simulink model "gm_PF"  (R2015a)
settings: Solver=FixedStepDiscrete  SolverMode=SingleTasking  StartTime=0.0  StopTime=2  RelTol=1e-3
libraries: dspsrcs4 x3, dspsnks4 x1
settings Model: Creator=aluno  LastModifiedBy=aluno
settings DataIOCC: SaveOutput=off  SaveTime=off
settings OptimizationCC: BlockReduction=off  ConditionallyExecuteInputs=off  InlineParams=on
settings DebuggingCC: AlgebraicLoopMsg=error  InheritedTsInSrcMsg=none  SingleTaskRateTransMsg=error  StrictBusMsg=ErrorOnBusTreatedAsVector
settings HardwareCC: ProdHWDeviceType=ASIC/FPGA->ASIC/FPGA  ProdEqTarget=off

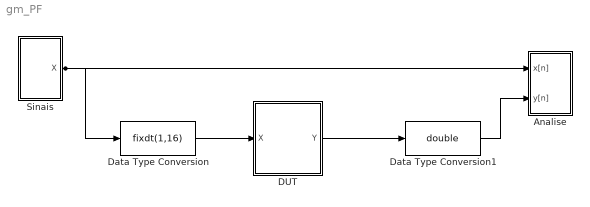
== system gm_PF ==
  Analise : Subsystem
  DUT : Subsystem
  Data Type Conversion : DataTypeConversion  OutMin=-1  OutMax=0.99  OutDataTypeStr=fixdt(1,16)
  Data Type Conversion1 : DataTypeConversion  OutDataTypeStr=double
  Sinais : Subsystem  mask{fa=8000, spf=1, fonte=2, v1=0.5, f1=1000, tchirp=2}
      mask prompts: fa "Freq. amostragem (Hz)"; spf "Amostras por frame"; fonte "Fonte (switch)"; v1 "Amplitude da senoide"; f1 "Freq. da senoide"; tchirp "Tempo Chirp"
      mask TypeOptions fonte: 1 | 2 | 3 | 4 | 5
  wires:
  Data Type Conversion1/1 -> Analise/2(y[n])
  Data Type Conversion/1 -> DUT/1(X)
  DUT/1(Y) -> Data Type Conversion1/1
  Sinais/1(X) -> Data Type Conversion/1, Analise/1(x[n])

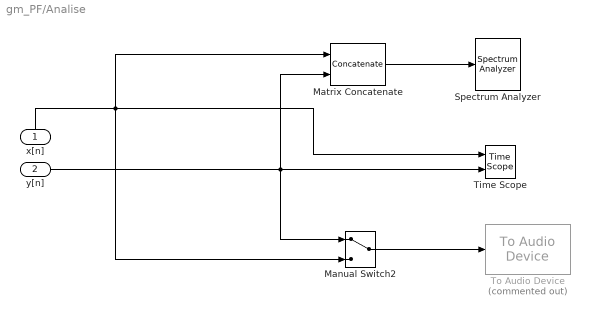
== system gm_PF/Analise ==
  x[n] : Inport
  y[n] : Inport  Port=2
  Manual Switch2 : ManualSwitch
  Matrix Concatenate : Concatenate  Mode=Multidimensional array  ConcatenateDimension=2
  Spectrum Analyzer : SpectrumAnalyzer
  Time Scope : TimeScope  DefaultConfigurationName=spbscopes.TimeScopeBlockCfg  NumInputPorts=2
  To Audio Device : dspsnks4/To Audio Device  Commented=on  deviceName=Default  inheritSampleRate=on  sampleRate=44100  deviceDatatype=Determine from input data type  autoBufferSize=on  bufferSize=4096  queueDuration=1.0  defaultOutputChannelMapping=on  outputChannelMapping=1:2  outputNumUnderrunSamples=off
  wires:
  Manual Switch2/1 -> To Audio Device/1
  y[n]/1 -> Time Scope/2, Matrix Concatenate/2, Manual Switch2/1
  x[n]/1 -> Matrix Concatenate/1, Time Scope/1, Manual Switch2/2
  Matrix Concatenate/1 -> Spectrum Analyzer/1

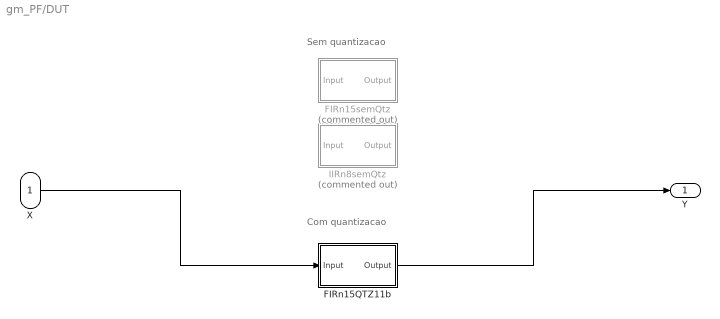
== system gm_PF/DUT ==
  note: Sem quantizacao
  note: Com quantizacao
  X : Inport
  FIRn15QTZ11b : Subsystem  Tag=FilterWizardSubSystem
      settings: ErrorFcn=dspFilterRealizedInBasicElemsAlgLoopErrFcnCallback
  FIRn15semQtz : Subsystem  Tag=FilterWizardSubSystem  Commented=on
      settings: ErrorFcn=dspFilterRealizedInBasicElemsAlgLoopErrFcnCallback
  IIRn8semQtz : Subsystem  Tag=FilterWizardSubSystem  Commented=on
      settings: ErrorFcn=dspFilterRealizedInBasicElemsAlgLoopErrFcnCallback
  Y : Outport
  wires:
  FIRn15QTZ11b/1(Output) -> Y/1
  X/1 -> FIRn15QTZ11b/1(Input)

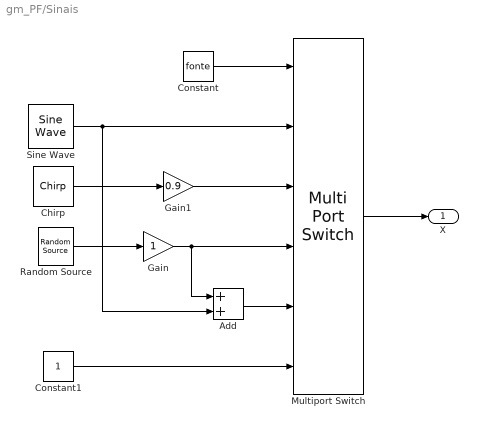
== system gm_PF/Sinais ==
  Add : Sum
  Chirp : dspsrcs4/Chirp  sweep=Linear  mode=Unidirectional  f0=1  f1=fa/2  t1=tchirp  Tsweep=tchirp  phase=0  Ts=1/fa  spf=spf  datatype=Double
  Constant : Constant  Value=fonte
  Constant1 : Constant
  Gain : Gain
  Gain1 : Gain  Gain=0.9
  Multiport Switch : MultiPortSwitch  Inputs=5
  Random Source : dspsrcs4/Random Source  SrcType=Uniform  NormMethod=Ziggurat  CltLength=12  MinVal=-1  MaxVal=1  MeanVal=0  VarVal=1  RepMode=Not repeatable  rawSeed=1  IsInherit=off  SampMode=Discrete  SampTime=1/fa  SampFrame=spf  DataType=Double  OutComplex=Real
  Sine Wave : dspsrcs4/Sine Wave  Amplitude=v1  Frequency=f1  Phase=0  SampleMode=Discrete  OutComplex=Real  CompMethod=Trigonometric fcn  TableSize=Speed  SampleTime=1/fa  SamplesPerFrame=spf  ResetState=Restart at time zero  dataType=double  wordLen=16  udDataType=sfix(16)  fracBitsMode=Best precision  numFracBits=15  OutDataTypeStr=double  LastOutDataTypeStr=double
  X : Outport
  wires:
  Gain1/1 -> Multiport Switch/3
  Random Source/1 -> Gain/1
  Constant1/1 -> Multiport Switch/6
  Add/1 -> Multiport Switch/5
  Constant/1 -> Multiport Switch/1
  Multiport Switch/1 -> X/1
  Sine Wave/1 -> Multiport Switch/2, Add/2
  Chirp/1 -> Gain1/1
  Gain/1 -> Multiport Switch/4, Add/1

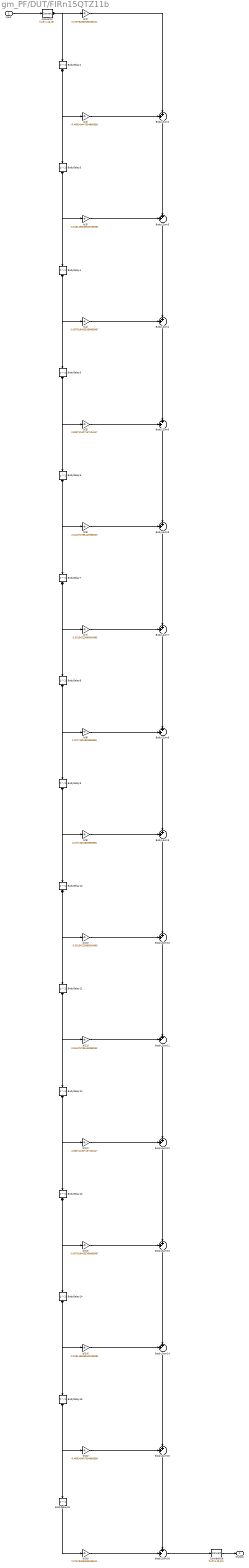
== system gm_PF/DUT/FIRn15QTZ11b ==
  Input : Inport
  BodyDelay{2..16} (15 alike) : Delay  DelayLength=1  InitialCondition=0
  BodyLSum{2..16} (15 alike) : Sum  Inputs=++|  AccumDataTypeStr=fixdt(1,28,23)  OutDataTypeStr=fixdt(1,28,23)  RndMeth=Convergent
  ConvertIn : DataTypeConversion  OutDataTypeStr=fixdt(1,16,15)  RndMeth=Nearest  SaturateOnIntegerOverflow=on
  ConvertOut : DataTypeConversion  OutDataTypeStr=fixdt(1,28,23)  RndMeth=Convergent
  b(1) : Gain  Gain=0.276784850536256011  ParamDataTypeStr=fixdt(1,11,8)  OutDataTypeStr=fixdt(1,26,23)  RndMeth=Convergent
  b(10) : Gain  Gain=-3.30154223899504995  ParamDataTypeStr=fixdt(1,11,8)  OutDataTypeStr=fixdt(1,26,23)  RndMeth=Convergent
  b(11) : Gain  Gain=0.514373785443998033  ParamDataTypeStr=fixdt(1,11,8)  OutDataTypeStr=fixdt(1,26,23)  RndMeth=Convergent
  b(12) : Gain  Gain=0.808711927137104047  ParamDataTypeStr=fixdt(1,11,8)  OutDataTypeStr=fixdt(1,26,23)  RndMeth=Convergent
  b(13) : Gain  Gain=-0.0579194055369869967  ParamDataTypeStr=fixdt(1,11,8)  OutDataTypeStr=fixdt(1,26,23)  RndMeth=Convergent
  b(14) : Gain  Gain=-0.0181458335529195991  ParamDataTypeStr=fixdt(1,11,8)  OutDataTypeStr=fixdt(1,26,23)  RndMeth=Convergent
  b(15) : Gain  Gain=-0.468249447094866988  ParamDataTypeStr=fixdt(1,11,8)  OutDataTypeStr=fixdt(1,26,23)  RndMeth=Convergent
  b(16) : Gain  Gain=0.276784850536256011  ParamDataTypeStr=fixdt(1,11,8)  OutDataTypeStr=fixdt(1,26,23)  RndMeth=Convergent
  b(2) : Gain  Gain=-0.468249447094866988  ParamDataTypeStr=fixdt(1,11,8)  OutDataTypeStr=fixdt(1,26,23)  RndMeth=Convergent
  b(3) : Gain  Gain=-0.0181458335529195991  ParamDataTypeStr=fixdt(1,11,8)  OutDataTypeStr=fixdt(1,26,23)  RndMeth=Convergent
  b(4) : Gain  Gain=-0.0579194055369869967  ParamDataTypeStr=fixdt(1,11,8)  OutDataTypeStr=fixdt(1,26,23)  RndMeth=Convergent
  b(5) : Gain  Gain=0.808711927137104047  ParamDataTypeStr=fixdt(1,11,8)  OutDataTypeStr=fixdt(1,26,23)  RndMeth=Convergent
  b(6) : Gain  Gain=0.514373785443998033  ParamDataTypeStr=fixdt(1,11,8)  OutDataTypeStr=fixdt(1,26,23)  RndMeth=Convergent
  b(7) : Gain  Gain=-3.30154223899504995  ParamDataTypeStr=fixdt(1,11,8)  OutDataTypeStr=fixdt(1,26,23)  RndMeth=Convergent
  b(8) : Gain  Gain=2.20774610833568996  ParamDataTypeStr=fixdt(1,11,8)  OutDataTypeStr=fixdt(1,26,23)  RndMeth=Convergent
  b(9) : Gain  Gain=2.20774610833568996  ParamDataTypeStr=fixdt(1,11,8)  OutDataTypeStr=fixdt(1,26,23)  RndMeth=Convergent
  Output : Outport
  wires:
  ConvertOut/1 -> Output/1
  BodyLSum16/1 -> ConvertOut/1
  b(16)/1 -> BodyLSum16/2
  BodyDelay16/1 -> b(16)/1
  BodyLSum15/1 -> BodyLSum16/1
  b(15)/1 -> BodyLSum15/1
  BodyDelay15/1 -> BodyDelay16/1, b(15)/1
  BodyLSum14/1 -> BodyLSum15/2
  b(14)/1 -> BodyLSum14/1
  BodyDelay14/1 -> BodyDelay15/1, b(14)/1
  BodyLSum13/1 -> BodyLSum14/2
  b(13)/1 -> BodyLSum13/1
  BodyDelay13/1 -> BodyDelay14/1, b(13)/1
  BodyLSum12/1 -> BodyLSum13/2
  b(12)/1 -> BodyLSum12/1
  BodyDelay12/1 -> BodyDelay13/1, b(12)/1
  BodyLSum11/1 -> BodyLSum12/2
  b(11)/1 -> BodyLSum11/1
  BodyDelay11/1 -> BodyDelay12/1, b(11)/1
  BodyLSum10/1 -> BodyLSum11/2
  b(10)/1 -> BodyLSum10/1
  BodyDelay10/1 -> BodyDelay11/1, b(10)/1
  BodyLSum9/1 -> BodyLSum10/2
  b(9)/1 -> BodyLSum9/1
  BodyDelay9/1 -> BodyDelay10/1, b(9)/1
  BodyLSum8/1 -> BodyLSum9/2
  b(8)/1 -> BodyLSum8/1
  BodyDelay8/1 -> BodyDelay9/1, b(8)/1
  BodyLSum7/1 -> BodyLSum8/2
  b(7)/1 -> BodyLSum7/1
  BodyDelay7/1 -> BodyDelay8/1, b(7)/1
  BodyLSum6/1 -> BodyLSum7/2
  b(6)/1 -> BodyLSum6/1
  BodyDelay6/1 -> BodyDelay7/1, b(6)/1
  BodyLSum5/1 -> BodyLSum6/2
  b(5)/1 -> BodyLSum5/1
  BodyDelay5/1 -> BodyDelay6/1, b(5)/1
  BodyLSum4/1 -> BodyLSum5/2
  b(4)/1 -> BodyLSum4/1
  BodyDelay4/1 -> BodyDelay5/1, b(4)/1
  BodyLSum3/1 -> BodyLSum4/2
  b(3)/1 -> BodyLSum3/1
  BodyDelay3/1 -> BodyDelay4/1, b(3)/1
  BodyLSum2/1 -> BodyLSum3/2
  b(2)/1 -> BodyLSum2/1
  BodyDelay2/1 -> BodyDelay3/1, b(2)/1
  ConvertIn/1 -> BodyDelay2/1, b(1)/1
  b(1)/1 -> BodyLSum2/2
  Input/1 -> ConvertIn/1

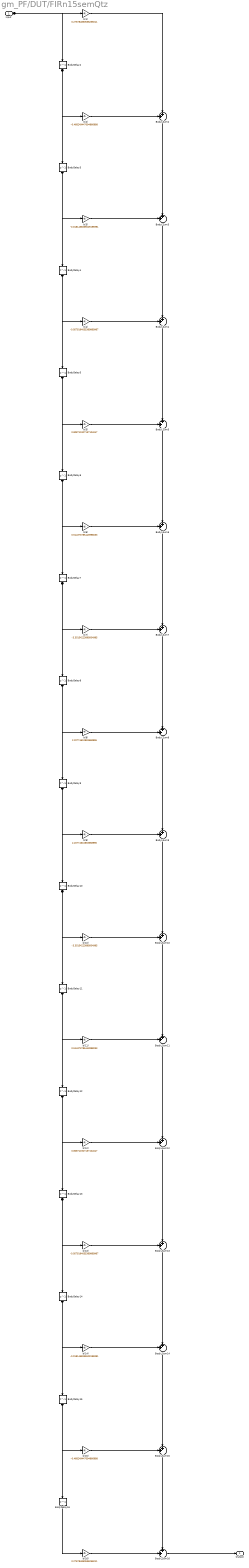
== system gm_PF/DUT/FIRn15semQtz ==
  Input : Inport
  BodyDelay{2..16} (15 alike) : Delay  DelayLength=1  InitialCondition=0  InputProcessing=Columns as channels (frame based)
  BodyLSum{2..16} (15 alike) : Sum  Inputs=++|  RndMeth=Nearest  SaturateOnIntegerOverflow=on  OutDataTypeStr=Inherit: Same as first input
  b(1) : Gain  Gain=0.276784850536256011  ParamDataTypeStr=double  RndMeth=Nearest  SaturateOnIntegerOverflow=on  OutDataTypeStr=Inherit: Same as input
  b(10) : Gain  Gain=-3.30154223899504995  ParamDataTypeStr=double  RndMeth=Nearest  SaturateOnIntegerOverflow=on  OutDataTypeStr=Inherit: Same as input
  b(11) : Gain  Gain=0.514373785443998033  ParamDataTypeStr=double  RndMeth=Nearest  SaturateOnIntegerOverflow=on  OutDataTypeStr=Inherit: Same as input
  b(12) : Gain  Gain=0.808711927137104047  ParamDataTypeStr=double  RndMeth=Nearest  SaturateOnIntegerOverflow=on  OutDataTypeStr=Inherit: Same as input
  b(13) : Gain  Gain=-0.0579194055369869967  ParamDataTypeStr=double  RndMeth=Nearest  SaturateOnIntegerOverflow=on  OutDataTypeStr=Inherit: Same as input
  b(14) : Gain  Gain=-0.0181458335529195991  ParamDataTypeStr=double  RndMeth=Nearest  SaturateOnIntegerOverflow=on  OutDataTypeStr=Inherit: Same as input
  b(15) : Gain  Gain=-0.468249447094866988  ParamDataTypeStr=double  RndMeth=Nearest  SaturateOnIntegerOverflow=on  OutDataTypeStr=Inherit: Same as input
  b(16) : Gain  Gain=0.276784850536256011  ParamDataTypeStr=double  RndMeth=Nearest  SaturateOnIntegerOverflow=on  OutDataTypeStr=Inherit: Same as input
  b(2) : Gain  Gain=-0.468249447094866988  ParamDataTypeStr=double  RndMeth=Nearest  SaturateOnIntegerOverflow=on  OutDataTypeStr=Inherit: Same as input
  b(3) : Gain  Gain=-0.0181458335529195991  ParamDataTypeStr=double  RndMeth=Nearest  SaturateOnIntegerOverflow=on  OutDataTypeStr=Inherit: Same as input
  b(4) : Gain  Gain=-0.0579194055369869967  ParamDataTypeStr=double  RndMeth=Nearest  SaturateOnIntegerOverflow=on  OutDataTypeStr=Inherit: Same as input
  b(5) : Gain  Gain=0.808711927137104047  ParamDataTypeStr=double  RndMeth=Nearest  SaturateOnIntegerOverflow=on  OutDataTypeStr=Inherit: Same as input
  b(6) : Gain  Gain=0.514373785443998033  ParamDataTypeStr=double  RndMeth=Nearest  SaturateOnIntegerOverflow=on  OutDataTypeStr=Inherit: Same as input
  b(7) : Gain  Gain=-3.30154223899504995  ParamDataTypeStr=double  RndMeth=Nearest  SaturateOnIntegerOverflow=on  OutDataTypeStr=Inherit: Same as input
  b(8) : Gain  Gain=2.20774610833568996  ParamDataTypeStr=double  RndMeth=Nearest  SaturateOnIntegerOverflow=on  OutDataTypeStr=Inherit: Same as input
  b(9) : Gain  Gain=2.20774610833568996  ParamDataTypeStr=double  RndMeth=Nearest  SaturateOnIntegerOverflow=on  OutDataTypeStr=Inherit: Same as input
  Output : Outport
  wires:
  BodyLSum16/1 -> Output/1
  b(16)/1 -> BodyLSum16/2
  BodyDelay16/1 -> b(16)/1
  BodyLSum15/1 -> BodyLSum16/1
  b(15)/1 -> BodyLSum15/1
  BodyDelay15/1 -> BodyDelay16/1, b(15)/1
  BodyLSum14/1 -> BodyLSum15/2
  b(14)/1 -> BodyLSum14/1
  BodyDelay14/1 -> BodyDelay15/1, b(14)/1
  BodyLSum13/1 -> BodyLSum14/2
  b(13)/1 -> BodyLSum13/1
  BodyDelay13/1 -> BodyDelay14/1, b(13)/1
  BodyLSum12/1 -> BodyLSum13/2
  b(12)/1 -> BodyLSum12/1
  BodyDelay12/1 -> BodyDelay13/1, b(12)/1
  BodyLSum11/1 -> BodyLSum12/2
  b(11)/1 -> BodyLSum11/1
  BodyDelay11/1 -> BodyDelay12/1, b(11)/1
  BodyLSum10/1 -> BodyLSum11/2
  b(10)/1 -> BodyLSum10/1
  BodyDelay10/1 -> BodyDelay11/1, b(10)/1
  BodyLSum9/1 -> BodyLSum10/2
  b(9)/1 -> BodyLSum9/1
  BodyDelay9/1 -> BodyDelay10/1, b(9)/1
  BodyLSum8/1 -> BodyLSum9/2
  b(8)/1 -> BodyLSum8/1
  BodyDelay8/1 -> BodyDelay9/1, b(8)/1
  BodyLSum7/1 -> BodyLSum8/2
  b(7)/1 -> BodyLSum7/1
  BodyDelay7/1 -> BodyDelay8/1, b(7)/1
  BodyLSum6/1 -> BodyLSum7/2
  b(6)/1 -> BodyLSum6/1
  BodyDelay6/1 -> BodyDelay7/1, b(6)/1
  BodyLSum5/1 -> BodyLSum6/2
  b(5)/1 -> BodyLSum5/1
  BodyDelay5/1 -> BodyDelay6/1, b(5)/1
  BodyLSum4/1 -> BodyLSum5/2
  b(4)/1 -> BodyLSum4/1
  BodyDelay4/1 -> BodyDelay5/1, b(4)/1
  BodyLSum3/1 -> BodyLSum4/2
  b(3)/1 -> BodyLSum3/1
  BodyDelay3/1 -> BodyDelay4/1, b(3)/1
  BodyLSum2/1 -> BodyLSum3/2
  b(2)/1 -> BodyLSum2/1
  BodyDelay2/1 -> BodyDelay3/1, b(2)/1
  b(1)/1 -> BodyLSum2/2
  Input/1 -> BodyDelay2/1, b(1)/1

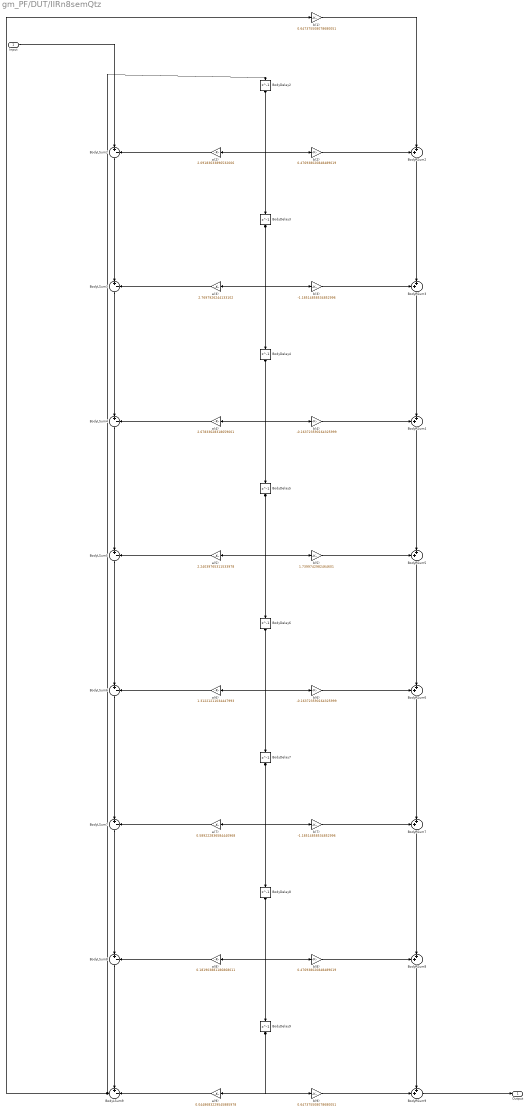
== system gm_PF/DUT/IIRn8semQtz ==
  Input : Inport
  BodyDelay{2..9} (8 alike) : Delay  DelayLength=1  InitialCondition=0
  BodyLSum{2..8} (7 alike) : Sum  Inputs=|+-  RndMeth=Nearest  SaturateOnIntegerOverflow=on  OutDataTypeStr=Inherit: Same as first input
  BodyLSum9 : Sum  Inputs=+-|  RndMeth=Nearest  SaturateOnIntegerOverflow=on  OutDataTypeStr=Inherit: Same as first input
  BodyRSum{2..9} (8 alike) : Sum  Inputs=++|  RndMeth=Nearest  SaturateOnIntegerOverflow=on  OutDataTypeStr=Inherit: Same as first input
  a(2) : Gain  Gain=2.09183633896532006  ParamDataTypeStr=double  RndMeth=Nearest  SaturateOnIntegerOverflow=on  OutDataTypeStr=Inherit: Same as input
  a(3) : Gain  Gain=2.7697926244133102  ParamDataTypeStr=double  RndMeth=Nearest  SaturateOnIntegerOverflow=on  OutDataTypeStr=Inherit: Same as input
  a(4) : Gain  Gain=2.67833628318659001  ParamDataTypeStr=double  RndMeth=Nearest  SaturateOnIntegerOverflow=on  OutDataTypeStr=Inherit: Same as input
  a(5) : Gain  Gain=2.24039765311533978  ParamDataTypeStr=double  RndMeth=Nearest  SaturateOnIntegerOverflow=on  OutDataTypeStr=Inherit: Same as input
  a(6) : Gain  Gain=1.31221211034447993  ParamDataTypeStr=double  RndMeth=Nearest  SaturateOnIntegerOverflow=on  OutDataTypeStr=Inherit: Same as input
  a(7) : Gain  Gain=0.589222836584440968  ParamDataTypeStr=double  RndMeth=Nearest  SaturateOnIntegerOverflow=on  OutDataTypeStr=Inherit: Same as input
  a(8) : Gain  Gain=0.181903881186868011  ParamDataTypeStr=double  RndMeth=Nearest  SaturateOnIntegerOverflow=on  OutDataTypeStr=Inherit: Same as input
  a(9) : Gain  Gain=0.0448683229545885978  ParamDataTypeStr=double  RndMeth=Nearest  SaturateOnIntegerOverflow=on  OutDataTypeStr=Inherit: Same as input
  b(1) : Gain  Gain=0.647375508078680051  ParamDataTypeStr=double  RndMeth=Nearest  SaturateOnIntegerOverflow=on  OutDataTypeStr=Inherit: Same as input
  b(2) : Gain  Gain=0.476938020848489019  ParamDataTypeStr=double  RndMeth=Nearest  SaturateOnIntegerOverflow=on  OutDataTypeStr=Inherit: Same as input
  b(3) : Gain  Gain=-1.18514858534852996  ParamDataTypeStr=double  RndMeth=Nearest  SaturateOnIntegerOverflow=on  OutDataTypeStr=Inherit: Same as input
  b(4) : Gain  Gain=-0.163723590164325999  ParamDataTypeStr=double  RndMeth=Nearest  SaturateOnIntegerOverflow=on  OutDataTypeStr=Inherit: Same as input
  b(5) : Gain  Gain=1.7399742982464601  ParamDataTypeStr=double  RndMeth=Nearest  SaturateOnIntegerOverflow=on  OutDataTypeStr=Inherit: Same as input
  b(6) : Gain  Gain=-0.163723590164325999  ParamDataTypeStr=double  RndMeth=Nearest  SaturateOnIntegerOverflow=on  OutDataTypeStr=Inherit: Same as input
  b(7) : Gain  Gain=-1.18514858534852996  ParamDataTypeStr=double  RndMeth=Nearest  SaturateOnIntegerOverflow=on  OutDataTypeStr=Inherit: Same as input
  b(8) : Gain  Gain=0.476938020848489019  ParamDataTypeStr=double  RndMeth=Nearest  SaturateOnIntegerOverflow=on  OutDataTypeStr=Inherit: Same as input
  b(9) : Gain  Gain=0.647375508078680051  ParamDataTypeStr=double  RndMeth=Nearest  SaturateOnIntegerOverflow=on  OutDataTypeStr=Inherit: Same as input
  Output : Outport
  wires:
  BodyRSum9/1 -> Output/1
  b(9)/1 -> BodyRSum9/2
  BodyDelay9/1 -> b(9)/1, a(9)/1
  a(9)/1 -> BodyLSum9/2
  BodyLSum9/1 -> BodyDelay2/1, b(1)/1
  BodyRSum8/1 -> BodyRSum9/1
  b(8)/1 -> BodyRSum8/1
  BodyDelay8/1 -> BodyDelay9/1, b(8)/1, a(8)/1
  a(8)/1 -> BodyLSum8/2
  BodyLSum8/1 -> BodyLSum9/1
  BodyRSum7/1 -> BodyRSum8/2
  b(7)/1 -> BodyRSum7/1
  BodyDelay7/1 -> BodyDelay8/1, b(7)/1, a(7)/1
  a(7)/1 -> BodyLSum7/2
  BodyLSum7/1 -> BodyLSum8/1
  BodyRSum6/1 -> BodyRSum7/2
  b(6)/1 -> BodyRSum6/1
  BodyDelay6/1 -> BodyDelay7/1, b(6)/1, a(6)/1
  a(6)/1 -> BodyLSum6/2
  BodyLSum6/1 -> BodyLSum7/1
  BodyRSum5/1 -> BodyRSum6/2
  b(5)/1 -> BodyRSum5/1
  BodyDelay5/1 -> BodyDelay6/1, b(5)/1, a(5)/1
  a(5)/1 -> BodyLSum5/2
  BodyLSum5/1 -> BodyLSum6/1
  BodyRSum4/1 -> BodyRSum5/2
  b(4)/1 -> BodyRSum4/1
  BodyDelay4/1 -> BodyDelay5/1, b(4)/1, a(4)/1
  a(4)/1 -> BodyLSum4/2
  BodyLSum4/1 -> BodyLSum5/1
  BodyRSum3/1 -> BodyRSum4/2
  b(3)/1 -> BodyRSum3/1
  BodyDelay3/1 -> BodyDelay4/1, b(3)/1, a(3)/1
  a(3)/1 -> BodyLSum3/2
  BodyLSum3/1 -> BodyLSum4/1
  BodyRSum2/1 -> BodyRSum3/2
  b(2)/1 -> BodyRSum2/1
  BodyDelay2/1 -> BodyDelay3/1, b(2)/1, a(2)/1
  a(2)/1 -> BodyLSum2/2
  BodyLSum2/1 -> BodyLSum3/1
  Input/1 -> BodyLSum2/1
  b(1)/1 -> BodyRSum2/2
